simulink model "CMOS_Kernel_Memory_Sync"  (R2023b)
settings: Solver=VariableStepAuto  StartTime=0.0  StopTime=30000000  RelTol=1e-3
values from neighbouring files (symbols this model uses):
  AmountOfPixelsPerScanline = 400    [Kernel_Setup_Script.m]
  AmountOfRamBlocksScanlines = 5    [Kernel_Setup_Script.m]
  AmountOfRamBlocksScanlinesOffset = AmountOfRamBlocksScanlines - 1    (= 4)    [Kernel_Setup_Script.m]
  AmountOfScanlinePixels = 73700    [Kernel_Setup_Script.m]
  AmountOfScanlinePixelsOffset = AmountOfScanlinePixels - 1    (= 73699)    [Kernel_Setup_Script.m]
  AmountOfScanlines = 1100    [Kernel_Setup_Script.m]
  AmountOfScanlinesOffset = AmountOfScanlines - 1    (= 1099)    [Kernel_Setup_Script.m]
  AOPPK_Off = AmountOfPixelsPerScanline - 1    (= 399)    [Kernel_Setup_Script.m]
  AOPPS_Off = AmountOfPixelsPerScanline - 1    (= 399)    [Kernel_Setup_Script.m]
  FramePackOff_0 = FramePackOff_0 - ScanlineFifoCheck    [Kernel_Setup_Script.m]
  FramePackOff_1 = FramePackOff_1 - ScanlineFifoCheck    [Kernel_Setup_Script.m]
  FramePackOff_2 = FramePackOff_2 - ScanlineFifoCheck    [Kernel_Setup_Script.m]
  FramePackOff_3 = FramePackOff_3 - ScanlineFifoCheck    [Kernel_Setup_Script.m]
  FramePackOff_4 = FramePackOff_4 - ScanlineFifoCheck    [Kernel_Setup_Script.m]
  FramePackOff_5 = FramePackOff_5 - ScanlineFifoCheck    [Kernel_Setup_Script.m]
  KernelPackOff_0 = KernelPackOff_0 - KernelBitsPerRow    [Kernel_Setup_Script.m]
  KernelPackOff_1 = KernelPackOff_1 - KernelBitsPerRow    [Kernel_Setup_Script.m]
  KernelPackOff_2 = KernelPackOff_2 - KernelBitsPerRow    [Kernel_Setup_Script.m]
  KernelPackOff_3 = KernelPackOff_3 - KernelBitsPerRow    [Kernel_Setup_Script.m]
  Slice59DownTo48Top = (MsbOffset - (ScanlinePixelBitSizeController*1))    (= 59)    [Kernel_Setup_Script.m]
  Slice71DownTo60Top = (MsbOffset - (ScanlinePixelBitSizeController*0))    (= 71)    [Kernel_Setup_Script.m]
  TotalSectionsForFrames = AmountOfScanlines/AmountOfRamBlocksScanlines    (= 220)    [Kernel_Setup_Script.m]
  UltraRamRows = AmountOfPixelsPerScanline/ScanlineFifoCheck    [Kernel_Setup_Script.m]
  UltraRamRowsCeil = ceil(AmountOfPixelsPerScanline/ScanlineFifoCheck)    [Kernel_Setup_Script.m]
  UltraRamRowsKernel = AmountOfPixelsPerScanline/KernelBitsPerRow    (= 100)    [Kernel_Setup_Script.m]
  UltraRamRowsKernelCeil = ceil(AmountOfPixelsPerScanline/KernelBitsPerRow)    [Kernel_Setup_Script.m]
  UltraRamRowsMemorySectionOffset = UltraRamRowsCeil*AmountOfRamBlocksScanlines    [Kernel_Setup_Script.m]
  UltraRamRowsOffset = UltraRamRowsCeil - 1    [Kernel_Setup_Script.m]
undefined symbols (not defined in the file or in its folder): c, Down, sfvc784, Up, xck26
libraries: hdlBasic x4512, vmcUtilities x1
(part 16 of 39)

== system CMOS_Kernel_Memory_Sync/Memory Handler/Data Slicer/Subsystem1/Delay Kernel Values RAM 2 ==
  Frame 12 Bit Bin Value 0 : Inport
  Frame 12 Bit Bin Value 1 : Inport  Port=2
  Frame 12 Bit Bin Value 2 : Inport  Port=3
  Frame 12 Bit Bin Value 3 : Inport  Port=4
  Frame 12 Bit Bin Value 4 : Inport  Port=5
  Frame 12 Bit Bin Value 5 : Inport  Port=6
  Frame 12 Bit Bin Value 6 : Inport  Port=7
  Frame 12 Bit Bin Value 7 : Inport  Port=8
  Frame 12 Bit Bin Value 8 : Inport  Port=9
  Frame 12 Bit Bin Value 9 : Inport  Port=10
  Frame 12 Bit Bin Value 10 : Inport  Port=11
  Frame 12 Bit Bin Value 11 : Inport  Port=12
  12 Bit Bin Value {0..23} (24 alike) : hdlBasic/Delay  rst=off  en=off  latency=1  reg_retiming=off  XmcBlockStatus=1  maskContainerNames=group1  block_type=delay  block_config=sysgen:Delay_config
  Kernel 18 Bit Value 0 : Outport
  Kernel 18 Bit Value 1 : Outport  Port=2
  Kernel 18 Bit Value 2 : Outport  Port=3
  Kernel 18 Bit Value 3 : Outport  Port=4
  Kernel 18 Bit Value 4 : Outport  Port=5
  Kernel 18 Bit Value 5 : Outport  Port=6
  Kernel 18 Bit Value 6 : Outport  Port=7
  Kernel 18 Bit Value 7 : Outport  Port=8
  Kernel 18 Bit Value 8 : Outport  Port=9
  Kernel 18 Bit Value 9 : Outport  Port=10
  Kernel 18 Bit Value 10 : Outport  Port=11
  Kernel 18 Bit Value 11 : Outport  Port=12
  wires:
  12 Bit Bin Value 2/1 -> Kernel 18 Bit Value 2/1
  Frame 12 Bit Bin Value 0/1 -> 12 Bit Bin Value 12/1
  Frame 12 Bit Bin Value 4/1 -> 12 Bit Bin Value 18/1
  12 Bit Bin Value 3/1 -> Kernel 18 Bit Value 3/1
  12 Bit Bin Value 0/1 -> Kernel 18 Bit Value 0/1
  Frame 12 Bit Bin Value 3/1 -> 12 Bit Bin Value 17/1
  Frame 12 Bit Bin Value 2/1 -> 12 Bit Bin Value 16/1
  12 Bit Bin Value 5/1 -> Kernel 18 Bit Value 5/1
  12 Bit Bin Value 4/1 -> Kernel 18 Bit Value 4/1
  Frame 12 Bit Bin Value 5/1 -> 12 Bit Bin Value 19/1
  12 Bit Bin Value 1/1 -> Kernel 18 Bit Value 1/1
  Frame 12 Bit Bin Value 1/1 -> 12 Bit Bin Value 13/1
  Frame 12 Bit Bin Value 7/1 -> 12 Bit Bin Value 21/1
  12 Bit Bin Value 11/1 -> Kernel 18 Bit Value 11/1
  12 Bit Bin Value 7/1 -> Kernel 18 Bit Value 7/1
  12 Bit Bin Value 10/1 -> Kernel 18 Bit Value 10/1
  Frame 12 Bit Bin Value 8/1 -> 12 Bit Bin Value 22/1
  Frame 12 Bit Bin Value 11/1 -> 12 Bit Bin Value 15/1
  Frame 12 Bit Bin Value 9/1 -> 12 Bit Bin Value 23/1
  12 Bit Bin Value 9/1 -> Kernel 18 Bit Value 9/1
  Frame 12 Bit Bin Value 6/1 -> 12 Bit Bin Value 20/1
  12 Bit Bin Value 6/1 -> Kernel 18 Bit Value 6/1
  12 Bit Bin Value 8/1 -> Kernel 18 Bit Value 8/1
  Frame 12 Bit Bin Value 10/1 -> 12 Bit Bin Value 14/1
  12 Bit Bin Value 13/1 -> 12 Bit Bin Value 1/1
  12 Bit Bin Value 14/1 -> 12 Bit Bin Value 10/1
  12 Bit Bin Value 15/1 -> 12 Bit Bin Value 11/1
  12 Bit Bin Value 16/1 -> 12 Bit Bin Value 2/1
  12 Bit Bin Value 17/1 -> 12 Bit Bin Value 3/1
  12 Bit Bin Value 19/1 -> 12 Bit Bin Value 5/1
  12 Bit Bin Value 18/1 -> 12 Bit Bin Value 4/1
  12 Bit Bin Value 23/1 -> 12 Bit Bin Value 9/1
  12 Bit Bin Value 21/1 -> 12 Bit Bin Value 7/1
  12 Bit Bin Value 20/1 -> 12 Bit Bin Value 6/1
  12 Bit Bin Value 22/1 -> 12 Bit Bin Value 8/1
  12 Bit Bin Value 12/1 -> 12 Bit Bin Value 0/1

== system CMOS_Kernel_Memory_Sync/Memory Handler/Data Slicer/Subsystem1/Delay Kernel Values RAM 3 ==
  Frame 12 Bit Bin Value 0 : Inport
  Frame 12 Bit Bin Value 1 : Inport  Port=2
  Frame 12 Bit Bin Value 2 : Inport  Port=3
  Frame 12 Bit Bin Value 3 : Inport  Port=4
  Frame 12 Bit Bin Value 4 : Inport  Port=5
  Frame 12 Bit Bin Value 5 : Inport  Port=6
  Frame 12 Bit Bin Value 6 : Inport  Port=7
  Frame 12 Bit Bin Value 7 : Inport  Port=8
  Frame 12 Bit Bin Value 8 : Inport  Port=9
  Frame 12 Bit Bin Value 9 : Inport  Port=10
  Frame 12 Bit Bin Value 10 : Inport  Port=11
  Frame 12 Bit Bin Value 11 : Inport  Port=12
  12 Bit Bin Value {0..23} (24 alike) : hdlBasic/Delay  rst=off  en=off  latency=1  reg_retiming=off  XmcBlockStatus=1  maskContainerNames=group1  block_type=delay  block_config=sysgen:Delay_config
  Kernel 18 Bit Value 0 : Outport
  Kernel 18 Bit Value 1 : Outport  Port=2
  Kernel 18 Bit Value 2 : Outport  Port=3
  Kernel 18 Bit Value 3 : Outport  Port=4
  Kernel 18 Bit Value 4 : Outport  Port=5
  Kernel 18 Bit Value 5 : Outport  Port=6
  Kernel 18 Bit Value 6 : Outport  Port=7
  Kernel 18 Bit Value 7 : Outport  Port=8
  Kernel 18 Bit Value 8 : Outport  Port=9
  Kernel 18 Bit Value 9 : Outport  Port=10
  Kernel 18 Bit Value 10 : Outport  Port=11
  Kernel 18 Bit Value 11 : Outport  Port=12
  wires:
  12 Bit Bin Value 2/1 -> Kernel 18 Bit Value 2/1
  Frame 12 Bit Bin Value 0/1 -> 12 Bit Bin Value 12/1
  Frame 12 Bit Bin Value 4/1 -> 12 Bit Bin Value 18/1
  12 Bit Bin Value 3/1 -> Kernel 18 Bit Value 3/1
  12 Bit Bin Value 0/1 -> Kernel 18 Bit Value 0/1
  Frame 12 Bit Bin Value 3/1 -> 12 Bit Bin Value 17/1
  Frame 12 Bit Bin Value 2/1 -> 12 Bit Bin Value 16/1
  12 Bit Bin Value 5/1 -> Kernel 18 Bit Value 5/1
  12 Bit Bin Value 4/1 -> Kernel 18 Bit Value 4/1
  Frame 12 Bit Bin Value 5/1 -> 12 Bit Bin Value 19/1
  12 Bit Bin Value 1/1 -> Kernel 18 Bit Value 1/1
  Frame 12 Bit Bin Value 1/1 -> 12 Bit Bin Value 13/1
  Frame 12 Bit Bin Value 7/1 -> 12 Bit Bin Value 21/1
  12 Bit Bin Value 11/1 -> Kernel 18 Bit Value 11/1
  12 Bit Bin Value 7/1 -> Kernel 18 Bit Value 7/1
  12 Bit Bin Value 10/1 -> Kernel 18 Bit Value 10/1
  Frame 12 Bit Bin Value 8/1 -> 12 Bit Bin Value 22/1
  Frame 12 Bit Bin Value 11/1 -> 12 Bit Bin Value 15/1
  Frame 12 Bit Bin Value 9/1 -> 12 Bit Bin Value 23/1
  12 Bit Bin Value 9/1 -> Kernel 18 Bit Value 9/1
  Frame 12 Bit Bin Value 6/1 -> 12 Bit Bin Value 20/1
  12 Bit Bin Value 6/1 -> Kernel 18 Bit Value 6/1
  12 Bit Bin Value 8/1 -> Kernel 18 Bit Value 8/1
  Frame 12 Bit Bin Value 10/1 -> 12 Bit Bin Value 14/1
  12 Bit Bin Value 13/1 -> 12 Bit Bin Value 1/1
  12 Bit Bin Value 14/1 -> 12 Bit Bin Value 10/1
  12 Bit Bin Value 15/1 -> 12 Bit Bin Value 11/1
  12 Bit Bin Value 16/1 -> 12 Bit Bin Value 2/1
  12 Bit Bin Value 17/1 -> 12 Bit Bin Value 3/1
  12 Bit Bin Value 19/1 -> 12 Bit Bin Value 5/1
  12 Bit Bin Value 18/1 -> 12 Bit Bin Value 4/1
  12 Bit Bin Value 23/1 -> 12 Bit Bin Value 9/1
  12 Bit Bin Value 21/1 -> 12 Bit Bin Value 7/1
  12 Bit Bin Value 20/1 -> 12 Bit Bin Value 6/1
  12 Bit Bin Value 22/1 -> 12 Bit Bin Value 8/1
  12 Bit Bin Value 12/1 -> 12 Bit Bin Value 0/1

== system CMOS_Kernel_Memory_Sync/Memory Handler/Data Slicer/Subsystem1/Delay Kernel Values RAM 4 ==
  Frame 12 Bit Bin Value 0 : Inport
  Frame 12 Bit Bin Value 1 : Inport  Port=2
  Frame 12 Bit Bin Value 2 : Inport  Port=3
  Frame 12 Bit Bin Value 3 : Inport  Port=4
  Frame 12 Bit Bin Value 4 : Inport  Port=5
  Frame 12 Bit Bin Value 5 : Inport  Port=6
  Frame 12 Bit Bin Value 6 : Inport  Port=7
  Frame 12 Bit Bin Value 7 : Inport  Port=8
  Frame 12 Bit Bin Value 8 : Inport  Port=9
  Frame 12 Bit Bin Value 9 : Inport  Port=10
  Frame 12 Bit Bin Value 10 : Inport  Port=11
  Frame 12 Bit Bin Value 11 : Inport  Port=12
  12 Bit Bin Value {0..23} (24 alike) : hdlBasic/Delay  rst=off  en=off  latency=1  reg_retiming=off  XmcBlockStatus=1  maskContainerNames=group1  block_type=delay  block_config=sysgen:Delay_config
  Kernel 18 Bit Value 0 : Outport
  Kernel 18 Bit Value 1 : Outport  Port=2
  Kernel 18 Bit Value 2 : Outport  Port=3
  Kernel 18 Bit Value 3 : Outport  Port=4
  Kernel 18 Bit Value 4 : Outport  Port=5
  Kernel 18 Bit Value 5 : Outport  Port=6
  Kernel 18 Bit Value 6 : Outport  Port=7
  Kernel 18 Bit Value 7 : Outport  Port=8
  Kernel 18 Bit Value 8 : Outport  Port=9
  Kernel 18 Bit Value 9 : Outport  Port=10
  Kernel 18 Bit Value 10 : Outport  Port=11
  Kernel 18 Bit Value 11 : Outport  Port=12
  wires:
  12 Bit Bin Value 2/1 -> Kernel 18 Bit Value 2/1
  Frame 12 Bit Bin Value 0/1 -> 12 Bit Bin Value 12/1
  Frame 12 Bit Bin Value 4/1 -> 12 Bit Bin Value 18/1
  12 Bit Bin Value 3/1 -> Kernel 18 Bit Value 3/1
  12 Bit Bin Value 0/1 -> Kernel 18 Bit Value 0/1
  Frame 12 Bit Bin Value 3/1 -> 12 Bit Bin Value 17/1
  Frame 12 Bit Bin Value 2/1 -> 12 Bit Bin Value 16/1
  12 Bit Bin Value 5/1 -> Kernel 18 Bit Value 5/1
  12 Bit Bin Value 4/1 -> Kernel 18 Bit Value 4/1
  Frame 12 Bit Bin Value 5/1 -> 12 Bit Bin Value 19/1
  12 Bit Bin Value 1/1 -> Kernel 18 Bit Value 1/1
  Frame 12 Bit Bin Value 1/1 -> 12 Bit Bin Value 13/1
  Frame 12 Bit Bin Value 7/1 -> 12 Bit Bin Value 21/1
  12 Bit Bin Value 11/1 -> Kernel 18 Bit Value 11/1
  12 Bit Bin Value 7/1 -> Kernel 18 Bit Value 7/1
  12 Bit Bin Value 10/1 -> Kernel 18 Bit Value 10/1
  Frame 12 Bit Bin Value 8/1 -> 12 Bit Bin Value 22/1
  Frame 12 Bit Bin Value 11/1 -> 12 Bit Bin Value 15/1
  Frame 12 Bit Bin Value 9/1 -> 12 Bit Bin Value 23/1
  12 Bit Bin Value 9/1 -> Kernel 18 Bit Value 9/1
  Frame 12 Bit Bin Value 6/1 -> 12 Bit Bin Value 20/1
  12 Bit Bin Value 6/1 -> Kernel 18 Bit Value 6/1
  12 Bit Bin Value 8/1 -> Kernel 18 Bit Value 8/1
  Frame 12 Bit Bin Value 10/1 -> 12 Bit Bin Value 14/1
  12 Bit Bin Value 13/1 -> 12 Bit Bin Value 1/1
  12 Bit Bin Value 14/1 -> 12 Bit Bin Value 10/1
  12 Bit Bin Value 15/1 -> 12 Bit Bin Value 11/1
  12 Bit Bin Value 16/1 -> 12 Bit Bin Value 2/1
  12 Bit Bin Value 17/1 -> 12 Bit Bin Value 3/1
  12 Bit Bin Value 19/1 -> 12 Bit Bin Value 5/1
  12 Bit Bin Value 18/1 -> 12 Bit Bin Value 4/1
  12 Bit Bin Value 23/1 -> 12 Bit Bin Value 9/1
  12 Bit Bin Value 21/1 -> 12 Bit Bin Value 7/1
  12 Bit Bin Value 20/1 -> 12 Bit Bin Value 6/1
  12 Bit Bin Value 22/1 -> 12 Bit Bin Value 8/1
  12 Bit Bin Value 12/1 -> 12 Bit Bin Value 0/1

== system CMOS_Kernel_Memory_Sync/Memory Handler/Data Slicer/Subsystem2/Delay Kernel Values RAM 0 ==
  Frame 12 Bit Bin Value 0 : Inport
  Frame 12 Bit Bin Value 1 : Inport  Port=2
  Frame 12 Bit Bin Value 2 : Inport  Port=3
  Frame 12 Bit Bin Value 3 : Inport  Port=4
  Frame 12 Bit Bin Value 4 : Inport  Port=5
  Frame 12 Bit Bin Value 5 : Inport  Port=6
  Frame 12 Bit Bin Value 6 : Inport  Port=7
  Frame 12 Bit Bin Value 7 : Inport  Port=8
  Frame 12 Bit Bin Value 8 : Inport  Port=9
  Frame 12 Bit Bin Value 9 : Inport  Port=10
  Frame 12 Bit Bin Value 10 : Inport  Port=11
  Frame 12 Bit Bin Value 11 : Inport  Port=12
  12 Bit Bin Value {0..23} (24 alike) : hdlBasic/Delay  rst=off  en=off  latency=1  reg_retiming=off  XmcBlockStatus=1  maskContainerNames=group1  block_type=delay  block_config=sysgen:Delay_config
  Kernel 18 Bit Value 0 : Outport
  Kernel 18 Bit Value 1 : Outport  Port=2
  Kernel 18 Bit Value 2 : Outport  Port=3
  Kernel 18 Bit Value 3 : Outport  Port=4
  Kernel 18 Bit Value 4 : Outport  Port=5
  Kernel 18 Bit Value 5 : Outport  Port=6
  Kernel 18 Bit Value 6 : Outport  Port=7
  Kernel 18 Bit Value 7 : Outport  Port=8
  Kernel 18 Bit Value 8 : Outport  Port=9
  Kernel 18 Bit Value 9 : Outport  Port=10
  Kernel 18 Bit Value 10 : Outport  Port=11
  Kernel 18 Bit Value 11 : Outport  Port=12
  wires:
  12 Bit Bin Value 2/1 -> Kernel 18 Bit Value 2/1
  Frame 12 Bit Bin Value 0/1 -> 12 Bit Bin Value 12/1
  Frame 12 Bit Bin Value 4/1 -> 12 Bit Bin Value 18/1
  12 Bit Bin Value 3/1 -> Kernel 18 Bit Value 3/1
  12 Bit Bin Value 0/1 -> Kernel 18 Bit Value 0/1
  Frame 12 Bit Bin Value 3/1 -> 12 Bit Bin Value 17/1
  Frame 12 Bit Bin Value 2/1 -> 12 Bit Bin Value 16/1
  12 Bit Bin Value 5/1 -> Kernel 18 Bit Value 5/1
  12 Bit Bin Value 4/1 -> Kernel 18 Bit Value 4/1
  Frame 12 Bit Bin Value 5/1 -> 12 Bit Bin Value 19/1
  12 Bit Bin Value 1/1 -> Kernel 18 Bit Value 1/1
  Frame 12 Bit Bin Value 1/1 -> 12 Bit Bin Value 13/1
  Frame 12 Bit Bin Value 7/1 -> 12 Bit Bin Value 21/1
  12 Bit Bin Value 11/1 -> Kernel 18 Bit Value 11/1
  12 Bit Bin Value 7/1 -> Kernel 18 Bit Value 7/1
  12 Bit Bin Value 10/1 -> Kernel 18 Bit Value 10/1
  Frame 12 Bit Bin Value 8/1 -> 12 Bit Bin Value 22/1
  Frame 12 Bit Bin Value 11/1 -> 12 Bit Bin Value 15/1
  Frame 12 Bit Bin Value 9/1 -> 12 Bit Bin Value 23/1
  12 Bit Bin Value 9/1 -> Kernel 18 Bit Value 9/1
  Frame 12 Bit Bin Value 6/1 -> 12 Bit Bin Value 20/1
  12 Bit Bin Value 6/1 -> Kernel 18 Bit Value 6/1
  12 Bit Bin Value 8/1 -> Kernel 18 Bit Value 8/1
  Frame 12 Bit Bin Value 10/1 -> 12 Bit Bin Value 14/1
  12 Bit Bin Value 13/1 -> 12 Bit Bin Value 1/1
  12 Bit Bin Value 14/1 -> 12 Bit Bin Value 10/1
  12 Bit Bin Value 15/1 -> 12 Bit Bin Value 11/1
  12 Bit Bin Value 16/1 -> 12 Bit Bin Value 2/1
  12 Bit Bin Value 17/1 -> 12 Bit Bin Value 3/1
  12 Bit Bin Value 19/1 -> 12 Bit Bin Value 5/1
  12 Bit Bin Value 18/1 -> 12 Bit Bin Value 4/1
  12 Bit Bin Value 23/1 -> 12 Bit Bin Value 9/1
  12 Bit Bin Value 21/1 -> 12 Bit Bin Value 7/1
  12 Bit Bin Value 20/1 -> 12 Bit Bin Value 6/1
  12 Bit Bin Value 22/1 -> 12 Bit Bin Value 8/1
  12 Bit Bin Value 12/1 -> 12 Bit Bin Value 0/1

== system CMOS_Kernel_Memory_Sync/Memory Handler/Data Slicer/Subsystem2/Delay Kernel Values RAM 1 ==
  Frame 12 Bit Bin Value 0 : Inport
  Frame 12 Bit Bin Value 1 : Inport  Port=2
  Frame 12 Bit Bin Value 2 : Inport  Port=3
  Frame 12 Bit Bin Value 3 : Inport  Port=4
  Frame 12 Bit Bin Value 4 : Inport  Port=5
  Frame 12 Bit Bin Value 5 : Inport  Port=6
  Frame 12 Bit Bin Value 6 : Inport  Port=7
  Frame 12 Bit Bin Value 7 : Inport  Port=8
  Frame 12 Bit Bin Value 8 : Inport  Port=9
  Frame 12 Bit Bin Value 9 : Inport  Port=10
  Frame 12 Bit Bin Value 10 : Inport  Port=11
  Frame 12 Bit Bin Value 11 : Inport  Port=12
  12 Bit Bin Value {0..23} (24 alike) : hdlBasic/Delay  rst=off  en=off  latency=1  reg_retiming=off  XmcBlockStatus=1  maskContainerNames=group1  block_type=delay  block_config=sysgen:Delay_config
  Kernel 18 Bit Value 0 : Outport
  Kernel 18 Bit Value 1 : Outport  Port=2
  Kernel 18 Bit Value 2 : Outport  Port=3
  Kernel 18 Bit Value 3 : Outport  Port=4
  Kernel 18 Bit Value 4 : Outport  Port=5
  Kernel 18 Bit Value 5 : Outport  Port=6
  Kernel 18 Bit Value 6 : Outport  Port=7
  Kernel 18 Bit Value 7 : Outport  Port=8
  Kernel 18 Bit Value 8 : Outport  Port=9
  Kernel 18 Bit Value 9 : Outport  Port=10
  Kernel 18 Bit Value 10 : Outport  Port=11
  Kernel 18 Bit Value 11 : Outport  Port=12
  wires:
  12 Bit Bin Value 2/1 -> Kernel 18 Bit Value 2/1
  Frame 12 Bit Bin Value 0/1 -> 12 Bit Bin Value 12/1
  Frame 12 Bit Bin Value 4/1 -> 12 Bit Bin Value 18/1
  12 Bit Bin Value 3/1 -> Kernel 18 Bit Value 3/1
  12 Bit Bin Value 0/1 -> Kernel 18 Bit Value 0/1
  Frame 12 Bit Bin Value 3/1 -> 12 Bit Bin Value 17/1
  Frame 12 Bit Bin Value 2/1 -> 12 Bit Bin Value 16/1
  12 Bit Bin Value 5/1 -> Kernel 18 Bit Value 5/1
  12 Bit Bin Value 4/1 -> Kernel 18 Bit Value 4/1
  Frame 12 Bit Bin Value 5/1 -> 12 Bit Bin Value 19/1
  12 Bit Bin Value 1/1 -> Kernel 18 Bit Value 1/1
  Frame 12 Bit Bin Value 1/1 -> 12 Bit Bin Value 13/1
  Frame 12 Bit Bin Value 7/1 -> 12 Bit Bin Value 21/1
  12 Bit Bin Value 11/1 -> Kernel 18 Bit Value 11/1
  12 Bit Bin Value 7/1 -> Kernel 18 Bit Value 7/1
  12 Bit Bin Value 10/1 -> Kernel 18 Bit Value 10/1
  Frame 12 Bit Bin Value 8/1 -> 12 Bit Bin Value 22/1
  Frame 12 Bit Bin Value 11/1 -> 12 Bit Bin Value 15/1
  Frame 12 Bit Bin Value 9/1 -> 12 Bit Bin Value 23/1
  12 Bit Bin Value 9/1 -> Kernel 18 Bit Value 9/1
  Frame 12 Bit Bin Value 6/1 -> 12 Bit Bin Value 20/1
  12 Bit Bin Value 6/1 -> Kernel 18 Bit Value 6/1
  12 Bit Bin Value 8/1 -> Kernel 18 Bit Value 8/1
  Frame 12 Bit Bin Value 10/1 -> 12 Bit Bin Value 14/1
  12 Bit Bin Value 13/1 -> 12 Bit Bin Value 1/1
  12 Bit Bin Value 14/1 -> 12 Bit Bin Value 10/1
  12 Bit Bin Value 15/1 -> 12 Bit Bin Value 11/1
  12 Bit Bin Value 16/1 -> 12 Bit Bin Value 2/1
  12 Bit Bin Value 17/1 -> 12 Bit Bin Value 3/1
  12 Bit Bin Value 19/1 -> 12 Bit Bin Value 5/1
  12 Bit Bin Value 18/1 -> 12 Bit Bin Value 4/1
  12 Bit Bin Value 23/1 -> 12 Bit Bin Value 9/1
  12 Bit Bin Value 21/1 -> 12 Bit Bin Value 7/1
  12 Bit Bin Value 20/1 -> 12 Bit Bin Value 6/1
  12 Bit Bin Value 22/1 -> 12 Bit Bin Value 8/1
  12 Bit Bin Value 12/1 -> 12 Bit Bin Value 0/1

== system CMOS_Kernel_Memory_Sync/Memory Handler/Data Slicer/Subsystem2/Delay Kernel Values RAM 2 ==
  Frame 12 Bit Bin Value 0 : Inport
  Frame 12 Bit Bin Value 1 : Inport  Port=2
  Frame 12 Bit Bin Value 2 : Inport  Port=3
  Frame 12 Bit Bin Value 3 : Inport  Port=4
  Frame 12 Bit Bin Value 4 : Inport  Port=5
  Frame 12 Bit Bin Value 5 : Inport  Port=6
  Frame 12 Bit Bin Value 6 : Inport  Port=7
  Frame 12 Bit Bin Value 7 : Inport  Port=8
  Frame 12 Bit Bin Value 8 : Inport  Port=9
  Frame 12 Bit Bin Value 9 : Inport  Port=10
  Frame 12 Bit Bin Value 10 : Inport  Port=11
  Frame 12 Bit Bin Value 11 : Inport  Port=12
  12 Bit Bin Value {0..23} (24 alike) : hdlBasic/Delay  rst=off  en=off  latency=1  reg_retiming=off  XmcBlockStatus=1  maskContainerNames=group1  block_type=delay  block_config=sysgen:Delay_config
  Kernel 18 Bit Value 0 : Outport
  Kernel 18 Bit Value 1 : Outport  Port=2
  Kernel 18 Bit Value 2 : Outport  Port=3
  Kernel 18 Bit Value 3 : Outport  Port=4
  Kernel 18 Bit Value 4 : Outport  Port=5
  Kernel 18 Bit Value 5 : Outport  Port=6
  Kernel 18 Bit Value 6 : Outport  Port=7
  Kernel 18 Bit Value 7 : Outport  Port=8
  Kernel 18 Bit Value 8 : Outport  Port=9
  Kernel 18 Bit Value 9 : Outport  Port=10
  Kernel 18 Bit Value 10 : Outport  Port=11
  Kernel 18 Bit Value 11 : Outport  Port=12
  wires:
  12 Bit Bin Value 2/1 -> Kernel 18 Bit Value 2/1
  Frame 12 Bit Bin Value 0/1 -> 12 Bit Bin Value 12/1
  Frame 12 Bit Bin Value 4/1 -> 12 Bit Bin Value 18/1
  12 Bit Bin Value 3/1 -> Kernel 18 Bit Value 3/1
  12 Bit Bin Value 0/1 -> Kernel 18 Bit Value 0/1
  Frame 12 Bit Bin Value 3/1 -> 12 Bit Bin Value 17/1
  Frame 12 Bit Bin Value 2/1 -> 12 Bit Bin Value 16/1
  12 Bit Bin Value 5/1 -> Kernel 18 Bit Value 5/1
  12 Bit Bin Value 4/1 -> Kernel 18 Bit Value 4/1
  Frame 12 Bit Bin Value 5/1 -> 12 Bit Bin Value 19/1
  12 Bit Bin Value 1/1 -> Kernel 18 Bit Value 1/1
  Frame 12 Bit Bin Value 1/1 -> 12 Bit Bin Value 13/1
  Frame 12 Bit Bin Value 7/1 -> 12 Bit Bin Value 21/1
  12 Bit Bin Value 11/1 -> Kernel 18 Bit Value 11/1
  12 Bit Bin Value 7/1 -> Kernel 18 Bit Value 7/1
  12 Bit Bin Value 10/1 -> Kernel 18 Bit Value 10/1
  Frame 12 Bit Bin Value 8/1 -> 12 Bit Bin Value 22/1
  Frame 12 Bit Bin Value 11/1 -> 12 Bit Bin Value 15/1
  Frame 12 Bit Bin Value 9/1 -> 12 Bit Bin Value 23/1
  12 Bit Bin Value 9/1 -> Kernel 18 Bit Value 9/1
  Frame 12 Bit Bin Value 6/1 -> 12 Bit Bin Value 20/1
  12 Bit Bin Value 6/1 -> Kernel 18 Bit Value 6/1
  12 Bit Bin Value 8/1 -> Kernel 18 Bit Value 8/1
  Frame 12 Bit Bin Value 10/1 -> 12 Bit Bin Value 14/1
  12 Bit Bin Value 13/1 -> 12 Bit Bin Value 1/1
  12 Bit Bin Value 14/1 -> 12 Bit Bin Value 10/1
  12 Bit Bin Value 15/1 -> 12 Bit Bin Value 11/1
  12 Bit Bin Value 16/1 -> 12 Bit Bin Value 2/1
  12 Bit Bin Value 17/1 -> 12 Bit Bin Value 3/1
  12 Bit Bin Value 19/1 -> 12 Bit Bin Value 5/1
  12 Bit Bin Value 18/1 -> 12 Bit Bin Value 4/1
  12 Bit Bin Value 23/1 -> 12 Bit Bin Value 9/1
  12 Bit Bin Value 21/1 -> 12 Bit Bin Value 7/1
  12 Bit Bin Value 20/1 -> 12 Bit Bin Value 6/1
  12 Bit Bin Value 22/1 -> 12 Bit Bin Value 8/1
  12 Bit Bin Value 12/1 -> 12 Bit Bin Value 0/1

== system CMOS_Kernel_Memory_Sync/Memory Handler/Data Slicer/Subsystem2/Delay Kernel Values RAM 3 ==
  Frame 12 Bit Bin Value 0 : Inport
  Frame 12 Bit Bin Value 1 : Inport  Port=2
  Frame 12 Bit Bin Value 2 : Inport  Port=3
  Frame 12 Bit Bin Value 3 : Inport  Port=4
  Frame 12 Bit Bin Value 4 : Inport  Port=5
  Frame 12 Bit Bin Value 5 : Inport  Port=6
  Frame 12 Bit Bin Value 6 : Inport  Port=7
  Frame 12 Bit Bin Value 7 : Inport  Port=8
  Frame 12 Bit Bin Value 8 : Inport  Port=9
  Frame 12 Bit Bin Value 9 : Inport  Port=10
  Frame 12 Bit Bin Value 10 : Inport  Port=11
  Frame 12 Bit Bin Value 11 : Inport  Port=12
  12 Bit Bin Value {0..23} (24 alike) : hdlBasic/Delay  rst=off  en=off  latency=1  reg_retiming=off  XmcBlockStatus=1  maskContainerNames=group1  block_type=delay  block_config=sysgen:Delay_config
  Kernel 18 Bit Value 0 : Outport
  Kernel 18 Bit Value 1 : Outport  Port=2
  Kernel 18 Bit Value 2 : Outport  Port=3
  Kernel 18 Bit Value 3 : Outport  Port=4
  Kernel 18 Bit Value 4 : Outport  Port=5
  Kernel 18 Bit Value 5 : Outport  Port=6
  Kernel 18 Bit Value 6 : Outport  Port=7
  Kernel 18 Bit Value 7 : Outport  Port=8
  Kernel 18 Bit Value 8 : Outport  Port=9
  Kernel 18 Bit Value 9 : Outport  Port=10
  Kernel 18 Bit Value 10 : Outport  Port=11
  Kernel 18 Bit Value 11 : Outport  Port=12
  wires:
  12 Bit Bin Value 2/1 -> Kernel 18 Bit Value 2/1
  Frame 12 Bit Bin Value 0/1 -> 12 Bit Bin Value 12/1
  Frame 12 Bit Bin Value 4/1 -> 12 Bit Bin Value 18/1
  12 Bit Bin Value 3/1 -> Kernel 18 Bit Value 3/1
  12 Bit Bin Value 0/1 -> Kernel 18 Bit Value 0/1
  Frame 12 Bit Bin Value 3/1 -> 12 Bit Bin Value 17/1
  Frame 12 Bit Bin Value 2/1 -> 12 Bit Bin Value 16/1
  12 Bit Bin Value 5/1 -> Kernel 18 Bit Value 5/1
  12 Bit Bin Value 4/1 -> Kernel 18 Bit Value 4/1
  Frame 12 Bit Bin Value 5/1 -> 12 Bit Bin Value 19/1
  12 Bit Bin Value 1/1 -> Kernel 18 Bit Value 1/1
  Frame 12 Bit Bin Value 1/1 -> 12 Bit Bin Value 13/1
  Frame 12 Bit Bin Value 7/1 -> 12 Bit Bin Value 21/1
  12 Bit Bin Value 11/1 -> Kernel 18 Bit Value 11/1
  12 Bit Bin Value 7/1 -> Kernel 18 Bit Value 7/1
  12 Bit Bin Value 10/1 -> Kernel 18 Bit Value 10/1
  Frame 12 Bit Bin Value 8/1 -> 12 Bit Bin Value 22/1
  Frame 12 Bit Bin Value 11/1 -> 12 Bit Bin Value 15/1
  Frame 12 Bit Bin Value 9/1 -> 12 Bit Bin Value 23/1
  12 Bit Bin Value 9/1 -> Kernel 18 Bit Value 9/1
  Frame 12 Bit Bin Value 6/1 -> 12 Bit Bin Value 20/1
  12 Bit Bin Value 6/1 -> Kernel 18 Bit Value 6/1
  12 Bit Bin Value 8/1 -> Kernel 18 Bit Value 8/1
  Frame 12 Bit Bin Value 10/1 -> 12 Bit Bin Value 14/1
  12 Bit Bin Value 13/1 -> 12 Bit Bin Value 1/1
  12 Bit Bin Value 14/1 -> 12 Bit Bin Value 10/1
  12 Bit Bin Value 15/1 -> 12 Bit Bin Value 11/1
  12 Bit Bin Value 16/1 -> 12 Bit Bin Value 2/1
  12 Bit Bin Value 17/1 -> 12 Bit Bin Value 3/1
  12 Bit Bin Value 19/1 -> 12 Bit Bin Value 5/1
  12 Bit Bin Value 18/1 -> 12 Bit Bin Value 4/1
  12 Bit Bin Value 23/1 -> 12 Bit Bin Value 9/1
  12 Bit Bin Value 21/1 -> 12 Bit Bin Value 7/1
  12 Bit Bin Value 20/1 -> 12 Bit Bin Value 6/1
  12 Bit Bin Value 22/1 -> 12 Bit Bin Value 8/1
  12 Bit Bin Value 12/1 -> 12 Bit Bin Value 0/1

== system CMOS_Kernel_Memory_Sync/Memory Handler/Data Slicer/Subsystem2/Delay Kernel Values RAM 4 ==
  Frame 12 Bit Bin Value 0 : Inport
  Frame 12 Bit Bin Value 1 : Inport  Port=2
  Frame 12 Bit Bin Value 2 : Inport  Port=3
  Frame 12 Bit Bin Value 3 : Inport  Port=4
  Frame 12 Bit Bin Value 4 : Inport  Port=5
  Frame 12 Bit Bin Value 5 : Inport  Port=6
  Frame 12 Bit Bin Value 6 : Inport  Port=7
  Frame 12 Bit Bin Value 7 : Inport  Port=8
  Frame 12 Bit Bin Value 8 : Inport  Port=9
  Frame 12 Bit Bin Value 9 : Inport  Port=10
  Frame 12 Bit Bin Value 10 : Inport  Port=11
  Frame 12 Bit Bin Value 11 : Inport  Port=12
  12 Bit Bin Value {0..23} (24 alike) : hdlBasic/Delay  rst=off  en=off  latency=1  reg_retiming=off  XmcBlockStatus=1  maskContainerNames=group1  block_type=delay  block_config=sysgen:Delay_config
  Kernel 18 Bit Value 0 : Outport
  Kernel 18 Bit Value 1 : Outport  Port=2
  Kernel 18 Bit Value 2 : Outport  Port=3
  Kernel 18 Bit Value 3 : Outport  Port=4
  Kernel 18 Bit Value 4 : Outport  Port=5
  Kernel 18 Bit Value 5 : Outport  Port=6
  Kernel 18 Bit Value 6 : Outport  Port=7
  Kernel 18 Bit Value 7 : Outport  Port=8
  Kernel 18 Bit Value 8 : Outport  Port=9
  Kernel 18 Bit Value 9 : Outport  Port=10
  Kernel 18 Bit Value 10 : Outport  Port=11
  Kernel 18 Bit Value 11 : Outport  Port=12
  wires:
  12 Bit Bin Value 2/1 -> Kernel 18 Bit Value 2/1
  Frame 12 Bit Bin Value 0/1 -> 12 Bit Bin Value 12/1
  Frame 12 Bit Bin Value 4/1 -> 12 Bit Bin Value 18/1
  12 Bit Bin Value 3/1 -> Kernel 18 Bit Value 3/1
  12 Bit Bin Value 0/1 -> Kernel 18 Bit Value 0/1
  Frame 12 Bit Bin Value 3/1 -> 12 Bit Bin Value 17/1
  Frame 12 Bit Bin Value 2/1 -> 12 Bit Bin Value 16/1
  12 Bit Bin Value 5/1 -> Kernel 18 Bit Value 5/1
  12 Bit Bin Value 4/1 -> Kernel 18 Bit Value 4/1
  Frame 12 Bit Bin Value 5/1 -> 12 Bit Bin Value 19/1
  12 Bit Bin Value 1/1 -> Kernel 18 Bit Value 1/1
  Frame 12 Bit Bin Value 1/1 -> 12 Bit Bin Value 13/1
  Frame 12 Bit Bin Value 7/1 -> 12 Bit Bin Value 21/1
  12 Bit Bin Value 11/1 -> Kernel 18 Bit Value 11/1
  12 Bit Bin Value 7/1 -> Kernel 18 Bit Value 7/1
  12 Bit Bin Value 10/1 -> Kernel 18 Bit Value 10/1
  Frame 12 Bit Bin Value 8/1 -> 12 Bit Bin Value 22/1
  Frame 12 Bit Bin Value 11/1 -> 12 Bit Bin Value 15/1
  Frame 12 Bit Bin Value 9/1 -> 12 Bit Bin Value 23/1
  12 Bit Bin Value 9/1 -> Kernel 18 Bit Value 9/1
  Frame 12 Bit Bin Value 6/1 -> 12 Bit Bin Value 20/1
  12 Bit Bin Value 6/1 -> Kernel 18 Bit Value 6/1
  12 Bit Bin Value 8/1 -> Kernel 18 Bit Value 8/1
  Frame 12 Bit Bin Value 10/1 -> 12 Bit Bin Value 14/1
  12 Bit Bin Value 13/1 -> 12 Bit Bin Value 1/1
  12 Bit Bin Value 14/1 -> 12 Bit Bin Value 10/1
  12 Bit Bin Value 15/1 -> 12 Bit Bin Value 11/1
  12 Bit Bin Value 16/1 -> 12 Bit Bin Value 2/1
  12 Bit Bin Value 17/1 -> 12 Bit Bin Value 3/1
  12 Bit Bin Value 19/1 -> 12 Bit Bin Value 5/1
  12 Bit Bin Value 18/1 -> 12 Bit Bin Value 4/1
  12 Bit Bin Value 23/1 -> 12 Bit Bin Value 9/1
  12 Bit Bin Value 21/1 -> 12 Bit Bin Value 7/1
  12 Bit Bin Value 20/1 -> 12 Bit Bin Value 6/1
  12 Bit Bin Value 22/1 -> 12 Bit Bin Value 8/1
  12 Bit Bin Value 12/1 -> 12 Bit Bin Value 0/1

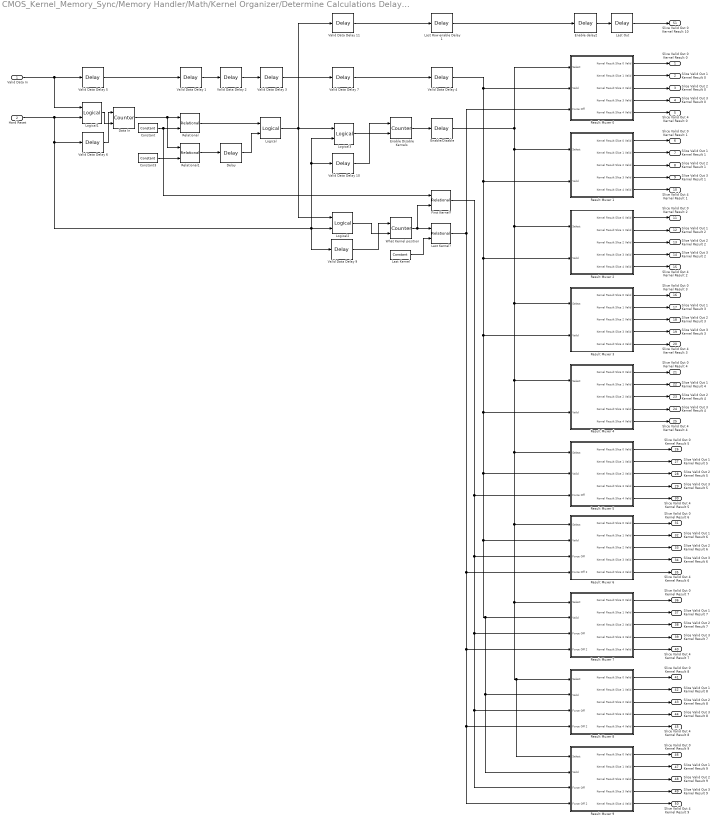
== system CMOS_Kernel_Memory_Sync/Memory Handler/Math/Kernel Organizer/Determine Calculations Delay 1 ==
  Valid Data In : Inport
  Hard Reset : Inport  Port=2
  Constant : hdlBasic/Constant  const=0  gui_display_data_type=Fixed-point  arith_type=Unsigned  n_bits=1  bin_pt=0  preci_type=Single  exp_width=8  frac_width=24  explicit_period=off  period=1  XmcBlockStatus=1  maskContainerNames=tabcontainer1  block_type=constant  block_config=sysgen:Constant_config
  Constant3 : hdlBasic/Constant  const=169  gui_display_data_type=Fixed-point  arith_type=Unsigned  n_bits=10  bin_pt=0  preci_type=Single  exp_width=8  frac_width=24  explicit_period=off  period=1  XmcBlockStatus=1  maskContainerNames=tabcontainer1  block_type=constant  block_config=sysgen:Constant_config
  Data In : hdlBasic/Counter  cnt_type=Count limited  cnt_to=169  operation=Up  start_count=0  cnt_by_val=1  arith_type=Unsigned  n_bits=10  bin_pt=0  load_pin=off  rst=on  en=on  explicit_period=Explicit  period=1  use_behavioral_HDL=off  implementation=Fabric  XmcBlockStatus=1  maskContainerNames=group1  block_type=counter  block_config=sysgen:Counter_config  block_width=531  block_height=1023
  Delay : hdlBasic/Delay  rst=off  en=off  latency=1  reg_retiming=off  XmcBlockStatus=1  maskContainerNames=group1  block_type=delay  block_config=sysgen:Delay_config
  Enable Disable Kernels : hdlBasic/Counter  cnt_type=Count limited  cnt_to=1  operation=Up  start_count=0  cnt_by_val=1  arith_type=Unsigned  n_bits=1  bin_pt=0  load_pin=off  rst=on  en=on  explicit_period=Explicit  period=1  use_behavioral_HDL=off  implementation=Fabric  XmcBlockStatus=1  maskContainerNames=group1  block_type=counter  block_config=sysgen:Counter_config  block_width=531  block_height=1023
  Enable delay2 : hdlBasic/Delay  rst=off  en=off  latency=1  reg_retiming=off  XmcBlockStatus=1  maskContainerNames=group1  block_type=delay  block_config=sysgen:Delay_config
  Enable/Disable : hdlBasic/Delay  rst=off  en=off  latency=1  reg_retiming=off  XmcBlockStatus=1  maskContainerNames=group1  block_type=delay  block_config=sysgen:Delay_config
  First Kernel? : hdlBasic/Relational  mode=a=b  op_type=Bool  en=off  latency=1  XmcBlockStatus=1  maskContainerNames=tabcontainer1  block_type=relational  block_config=sysgen:Relational_config
  Last Kernel : hdlBasic/Constant  const=219  gui_display_data_type=Fixed-point  arith_type=Unsigned  n_bits=10  bin_pt=0  preci_type=Single  exp_width=8  frac_width=24  explicit_period=off  period=1  XmcBlockStatus=1  maskContainerNames=tabcontainer1  block_type=constant  block_config=sysgen:Constant_config
  Last Kernel? : hdlBasic/Relational  mode=a=b  op_type=Bool  en=off  latency=1  XmcBlockStatus=1  maskContainerNames=tabcontainer1  block_type=relational  block_config=sysgen:Relational_config
  Last Out : hdlBasic/Delay  rst=off  en=off  latency=1  reg_retiming=off  XmcBlockStatus=1  maskContainerNames=group1  block_type=delay  block_config=sysgen:Delay_config
  Last Row enable Delay 1 : hdlBasic/Delay  rst=off  en=off  latency=1  reg_retiming=off  XmcBlockStatus=1  maskContainerNames=group1  block_type=delay  block_config=sysgen:Delay_config
  Logical : hdlBasic/Logical  logical_function=AND  inputs=2  en=off  latency=1  precision=Full  arith_type=Unsigned  n_bits=16  bin_pt=0  align_bp=on  overflow=[]  quantization=[]  XmcBlockStatus=1  maskContainerNames=tabcontainer1  block_type=logical  block_config=sysgen:Logical_config
  Logical1 : hdlBasic/Logical  logical_function=OR  inputs=2  en=off  latency=1  precision=Full  arith_type=Unsigned  n_bits=16  bin_pt=0  align_bp=on  overflow=[]  quantization=[]  XmcBlockStatus=1  maskContainerNames=tabcontainer1  block_type=logical  block_config=sysgen:Logical_config
  Logical2 : hdlBasic/Logical  logical_function=OR  inputs=2  en=off  latency=1  precision=Full  arith_type=Unsigned  n_bits=16  bin_pt=0  align_bp=on  overflow=[]  quantization=[]  XmcBlockStatus=1  maskContainerNames=tabcontainer1  block_type=logical  block_config=sysgen:Logical_config
  Logical3 : hdlBasic/Logical  logical_function=OR  inputs=2  en=off  latency=1  precision=Full  arith_type=Unsigned  n_bits=16  bin_pt=0  align_bp=on  overflow=[]  quantization=[]  XmcBlockStatus=1  maskContainerNames=tabcontainer1  block_type=logical  block_config=sysgen:Logical_config
  Relational : hdlBasic/Relational  mode=a=b  op_type=Bool  en=off  latency=1  XmcBlockStatus=1  maskContainerNames=tabcontainer1  block_type=relational  block_config=sysgen:Relational_config
  Relational1 : hdlBasic/Relational  mode=a=b  op_type=Bool  en=off  latency=1  XmcBlockStatus=1  maskContainerNames=tabcontainer1  block_type=relational  block_config=sysgen:Relational_config
  Result Muxer 0 : Subsystem
  Result Muxer 1 : Subsystem
  Result Muxer 2 : Subsystem
  Result Muxer 3 : Subsystem
  Result Muxer 4 : Subsystem
  Result Muxer 5 : Subsystem
  Result Muxer 6 : Subsystem
  Result Muxer 7 : Subsystem
  Result Muxer 8 : Subsystem
  Result Muxer 9 : Subsystem
  Valid Data Delay {1..7,9..11} (10 alike) : hdlBasic/Delay  rst=off  en=off  latency=1  reg_retiming=off  XmcBlockStatus=1  maskContainerNames=group1  block_type=delay  block_config=sysgen:Delay_config
  What Kernel position : hdlBasic/Counter  cnt_type=Count limited  cnt_to=219  operation=Up  start_count=0  cnt_by_val=1  arith_type=Unsigned  n_bits=12  bin_pt=0  load_pin=off  rst=on  en=on  explicit_period=Explicit  period=1  use_behavioral_HDL=off  implementation=Fabric  XmcBlockStatus=1  maskContainerNames=group1  block_type=counter  block_config=sysgen:Counter_config  block_width=531  block_height=1023
  Slice Valid Out 0 Kernel Result 0 : Outport
  Slice Valid Out 1 Kernel Result 0 : Outport  Port=2
  Slice Valid Out 2 Kernel Result 0 : Outport  Port=3
  Slice Valid Out 3 Kernel Result 0 : Outport  Port=4
  Slice Valid Out 4 Kernel Result 0 : Outport  Port=5
  Slice Valid Out 0 Kernel Result 1 : Outport  Port=6
  Slice Valid Out 1 Kernel Result 1 : Outport  Port=7
  Slice Valid Out 2 Kernel Result 1 : Outport  Port=8
  Slice Valid Out 3 Kernel Result 1 : Outport  Port=9
  Slice Valid Out 4 Kernel Result 1 : Outport  Port=10
  Slice Valid Out 0 Kernel Result 2 : Outport  Port=11
  Slice Valid Out 1 Kernel Result 2 : Outport  Port=12
  Slice Valid Out 2 Kernel Result 2 : Outport  Port=13
  Slice Valid Out 3 Kernel Result 2 : Outport  Port=14
  Slice Valid Out 4 Kernel Result 2 : Outport  Port=15
  Slice Valid Out 0 Kernel Result 3 : Outport  Port=16
  Slice Valid Out 1 Kernel Result 3 : Outport  Port=17
  Slice Valid Out 2 Kernel Result 3 : Outport  Port=18
  Slice Valid Out 3 Kernel Result 3 : Outport  Port=19
  Slice Valid Out 4 Kernel Result 3 : Outport  Port=20
  Slice Valid Out 0 Kernel Result 4 : Outport  Port=21
  Slice Valid Out 1 Kernel Result 4 : Outport  Port=22
  Slice Valid Out 2 Kernel Result 4 : Outport  Port=23
  Slice Valid Out 3 Kernel Result 4 : Outport  Port=24
  Slice Valid Out 4 Kernel Result 4 : Outport  Port=25
  Slice Valid Out 0 Kernel Result 5 : Outport  Port=26
  Slice Valid Out 1 Kernel Result 5 : Outport  Port=27
  Slice Valid Out 2 Kernel Result 5 : Outport  Port=28
  Slice Valid Out 3 Kernel Result 5 : Outport  Port=29
  Slice Valid Out 4 Kernel Result 5 : Outport  Port=30
  Slice Valid Out 0 Kernel Result 6 : Outport  Port=31
  Slice Valid Out 1 Kernel Result 6 : Outport  Port=32
  Slice Valid Out 2 Kernel Result 6 : Outport  Port=33
  Slice Valid Out 3 Kernel Result 6 : Outport  Port=34
  Slice Valid Out 4 Kernel Result 6 : Outport  Port=35
  Slice Valid Out 0 Kernel Result 7 : Outport  Port=36
  Slice Valid Out 1 Kernel Result 7 : Outport  Port=37
  Slice Valid Out 2 Kernel Result 7 : Outport  Port=38
  Slice Valid Out 3 Kernel Result 7 : Outport  Port=39
  Slice Valid Out 4 Kernel Result 7 : Outport  Port=40
  Slice Valid Out 0 Kernel Result 8 : Outport  Port=41
  Slice Valid Out 1 Kernel Result 8 : Outport  Port=42
  Slice Valid Out 2 Kernel Result 8 : Outport  Port=43
  Slice Valid Out 3 Kernel Result 8 : Outport  Port=44
  Slice Valid Out 4 Kernel Result 8 : Outport  Port=45
  Slice Valid Out 0 Kernel Result 9 : Outport  Port=46
  Slice Valid Out 1 Kernel Result 9 : Outport  Port=47
  Slice Valid Out 2 Kernel Result 9 : Outport  Port=48
  Slice Valid Out 3 Kernel Result 9 : Outport  Port=49
  Slice Valid Out 4 Kernel Result 9 : Outport  Port=50
  Slice Valid Out 0 Kernel Result 10 : Outport  Port=51
  wires:
  Valid Data In/1 -> Valid Data Delay 5/1, Logical1/1
  Result Muxer 0/3(Kernel Result Slice 2 Valid) -> Slice Valid Out 2 Kernel Result 0/1
  Result Muxer 0/5(Kernel Result Slice 4 Valid) -> Slice Valid Out 4 Kernel Result 0/1
  Result Muxer 0/2(Kernel Result Slice 1 Valid) -> Slice Valid Out 1 Kernel Result 0/1
  Result Muxer 0/1(Kernel Result Slice 0 Valid) -> Slice Valid Out 0 Kernel Result 0/1
  Result Muxer 0/4(Kernel Result Slice 3 Valid) -> Slice Valid Out 3 Kernel Result 0/1
  Result Muxer 1/5(Kernel Result Slice 4 Valid) -> Slice Valid Out 4 Kernel Result 1/1
  Result Muxer 1/2(Kernel Result Slice 1 Valid) -> Slice Valid Out 1 Kernel Result 1/1
  Result Muxer 1/4(Kernel Result Slice 3 Valid) -> Slice Valid Out 3 Kernel Result 1/1
  Result Muxer 1/3(Kernel Result Slice 2 Valid) -> Slice Valid Out 2 Kernel Result 1/1
  Result Muxer 1/1(Kernel Result Slice 0 Valid) -> Slice Valid Out 0 Kernel Result 1/1
  Result Muxer 2/3(Kernel Result Slice 2 Valid) -> Slice Valid Out 2 Kernel Result 2/1
  Result Muxer 2/1(Kernel Result Slice 0 Valid) -> Slice Valid Out 0 Kernel Result 2/1
  Result Muxer 2/4(Kernel Result Slice 3 Valid) -> Slice Valid Out 3 Kernel Result 2/1
  Result Muxer 2/5(Kernel Result Slice 4 Valid) -> Slice Valid Out 4 Kernel Result 2/1
  Result Muxer 2/2(Kernel Result Slice 1 Valid) -> Slice Valid Out 1 Kernel Result 2/1
  Result Muxer 3/2(Kernel Result Slice 1 Valid) -> Slice Valid Out 1 Kernel Result 3/1
  Result Muxer 3/5(Kernel Result Slice 4 Valid) -> Slice Valid Out 4 Kernel Result 3/1
  Result Muxer 3/4(Kernel Result Slice 3 Valid) -> Slice Valid Out 3 Kernel Result 3/1
  Result Muxer 3/1(Kernel Result Slice 0 Valid) -> Slice Valid Out 0 Kernel Result 3/1
  Result Muxer 3/3(Kernel Result Slice 2 Valid) -> Slice Valid Out 2 Kernel Result 3/1
  Result Muxer 4/4(Kernel Result Slice 3 Valid) -> Slice Valid Out 3 Kernel Result 4/1
  Result Muxer 4/2(Kernel Result Slice 1 Valid) -> Slice Valid Out 1 Kernel Result 4/1
  Result Muxer 4/5(Kernel Result Slice 4 Valid) -> Slice Valid Out 4 Kernel Result 4/1
  Result Muxer 4/3(Kernel Result Slice 2 Valid) -> Slice Valid Out 2 Kernel Result 4/1
  Result Muxer 4/1(Kernel Result Slice 0 Valid) -> Slice Valid Out 0 Kernel Result 4/1
  Constant3/1 -> Relational1/2
  Relational1/1 -> Delay/1
  Data In/1 -> Relational1/1, Relational/1
  Delay/1 -> Logical/2
  Relational/1 -> Logical/1
  Logical/1 -> Valid Data Delay 11/1, Logical2/1, Logical3/1
  Valid Data Delay 1/1 -> Valid Data Delay 2/1
  Valid Data Delay 2/1 -> Valid Data Delay 3/1
  Result Muxer 5/2(Kernel Result Slice 1 Valid) -> Slice Valid Out 1 Kernel Result 5/1
  Result Muxer 5/5(Kernel Result Slice 4 Valid) -> Slice Valid Out 4 Kernel Result 5/1
  Result Muxer 5/1(Kernel Result Slice 0 Valid) -> Slice Valid Out 0 Kernel Result 5/1
  Result Muxer 5/4(Kernel Result Slice 3 Valid) -> Slice Valid Out 3 Kernel Result 5/1
  Result Muxer 5/3(Kernel Result Slice 2 Valid) -> Slice Valid Out 2 Kernel Result 5/1
  Result Muxer 6/1(Kernel Result Slice 0 Valid) -> Slice Valid Out 0 Kernel Result 6/1
  Result Muxer 6/4(Kernel Result Slice 3 Valid) -> Slice Valid Out 3 Kernel Result 6/1
  Result Muxer 6/5(Kernel Result Slice 4 Valid) -> Slice Valid Out 4 Kernel Result 6/1
  Result Muxer 6/3(Kernel Result Slice 2 Valid) -> Slice Valid Out 2 Kernel Result 6/1
  Result Muxer 6/2(Kernel Result Slice 1 Valid) -> Slice Valid Out 1 Kernel Result 6/1
  Result Muxer 7/1(Kernel Result Slice 0 Valid) -> Slice Valid Out 0 Kernel Result 7/1
  Result Muxer 7/4(Kernel Result Slice 3 Valid) -> Slice Valid Out 3 Kernel Result 7/1
  Result Muxer 7/5(Kernel Result Slice 4 Valid) -> Slice Valid Out 4 Kernel Result 7/1
  Result Muxer 7/3(Kernel Result Slice 2 Valid) -> Slice Valid Out 2 Kernel Result 7/1
  Result Muxer 7/2(Kernel Result Slice 1 Valid) -> Slice Valid Out 1 Kernel Result 7/1
  Result Muxer 8/1(Kernel Result Slice 0 Valid) -> Slice Valid Out 0 Kernel Result 8/1
  Result Muxer 8/4(Kernel Result Slice 3 Valid) -> Slice Valid Out 3 Kernel Result 8/1
  Result Muxer 8/5(Kernel Result Slice 4 Valid) -> Slice Valid Out 4 Kernel Result 8/1
  Result Muxer 8/3(Kernel Result Slice 2 Valid) -> Slice Valid Out 2 Kernel Result 8/1
  Result Muxer 8/2(Kernel Result Slice 1 Valid) -> Slice Valid Out 1 Kernel Result 8/1
  Result Muxer 9/1(Kernel Result Slice 0 Valid) -> Slice Valid Out 0 Kernel Result 9/1
  Result Muxer 9/4(Kernel Result Slice 3 Valid) -> Slice Valid Out 3 Kernel Result 9/1
  Result Muxer 9/5(Kernel Result Slice 4 Valid) -> Slice Valid Out 4 Kernel Result 9/1
  Result Muxer 9/3(Kernel Result Slice 2 Valid) -> Slice Valid Out 2 Kernel Result 9/1
  Result Muxer 9/2(Kernel Result Slice 1 Valid) -> Slice Valid Out 1 Kernel Result 9/1
  Last Kernel/1 -> Last Kernel?/2
  What Kernel position/1 -> First Kernel?/2, Last Kernel?/1
  First Kernel?/1 -> Result Muxer 5/3(Force Off), Result Muxer 7/3(Force Off), Result Muxer 8/3(Force Off), Result Muxer 9/3(Force Off), Result Muxer 6/3(Force Off)
  Last Kernel?/1 -> Result Muxer 0/3(Force Off), Result Muxer 6/4(Force Off 2), Result Muxer 7/4(Force Off 2), Result Muxer 8/4(Force Off 2), Result Muxer 9/4(Force Off 2)
  Enable Disable Kernels/1 -> Enable/Disable/1
  Valid Data Delay 3/1 -> Valid Data Delay 7/1
  Enable/Disable/1 -> Result Muxer 0/1(Select), Result Muxer 9/1(Select), Result Muxer 8/1(Select), Result Muxer 7/1(Select), Result Muxer 6/1(Select), Result Muxer 5/1(Select), Result Muxer 4/1(Select), Result Muxer 3/1(Select), Result Muxer 2/1(Select), Result Muxer 1/1(Select)
  Valid Data Delay 4/1 -> Result Muxer 9/2(Valid), Result Muxer 8/2(Valid), Result Muxer 7/2(Valid), Result Muxer 6/2(Valid), Result Muxer 5/2(Valid), Result Muxer 4/2(Valid), Result Muxer 3/2(Valid), Result Muxer 2/2(Valid), Result Muxer 1/2(Valid), Result Muxer 0/2(Valid)
  Enable delay2/1 -> Last Out/1
  Last Row enable Delay 1/1 -> Enable delay2/1
  Last Out/1 -> Slice Valid Out 0 Kernel Result 10/1
  Valid Data Delay 5/1 -> Valid Data Delay 1/1
  Hard Reset/1 -> Logical1/2, Valid Data Delay 9/1, Valid Data Delay 10/1, Logical3/2, Logical2/2, Valid Data Delay 6/1
  Valid Data Delay 6/1 -> Data In/1
  Valid Data Delay 7/1 -> Valid Data Delay 4/1
  Constant/1 -> First Kernel?/1, Relational/2
  Logical2/1 -> What Kernel position/2
  Valid Data Delay 9/1 -> What Kernel position/1
  Logical3/1 -> Enable Disable Kernels/2
  Valid Data Delay 10/1 -> Enable Disable Kernels/1
  Valid Data Delay 11/1 -> Last Row enable Delay 1/1
  Logical1/1 -> Data In/2
